simulink model "cruisecontrolsystem"  (R2020b)
settings: Solver=VariableStepAuto  StartTime=0.0  StopTime=120.0  RelTol=1e-3
PreLoadFcn:
  | clear all;
  | close all;
  | clc;
  | m=1000;
  | b=50;
  | u=500;
settings Model: DataDictionary=Data.sldd  Creator=Admin  LastModifiedBy=Admin

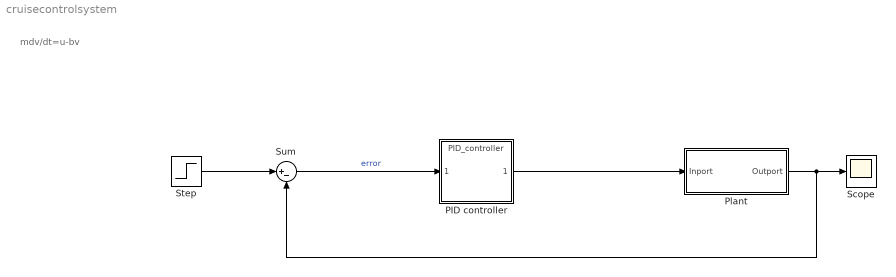
== system cruisecontrolsystem ==
  note: mdv/dt=u-bv
  PID controller : ModelReference  ModelNameDialog=PID_controller  SimulationMode=Normal  ModelReferenceVersion=1.17
  Plant : Subsystem
  Scope : Scope
  Step : Step  Time=0  After=u  SampleTime=0
  Sum : Sum  Inputs=|+-
  wires:
  Plant/1(Outport) -> Sum/2, Scope/1
  PID controller/1 -> Plant/1(Inport)
  Step/1 -> Sum/1
  Sum/1 -> PID controller/1  "error"

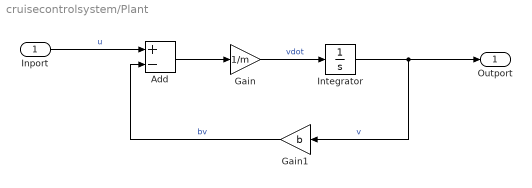
== system cruisecontrolsystem/Plant ==
  Inport : Inport
  Add : Sum  Inputs=+-
  Gain : Gain  Gain=1/m
  Gain1 : Gain  Gain=b
  Integrator : Integrator
  Outport : Outport
  wires:
  Gain1/1 -> Add/2  "bv"
  Add/1 -> Gain/1
  Integrator/1 -> Outport/1, Gain1/1  "v"
  Gain/1 -> Integrator/1  "vdot"
  Inport/1 -> Add/1  "u"
